simulink model "PFC_V11"  (R2016b)
settings: Solver=FixedStepDiscrete  StartTime=0.0  StopTime=0.1  FixedStep=.1e-6  RelTol=1e-3
libraries: powerlib x29, simulink x5
settings Model: Creator=a037702  LastModifiedBy=a037702

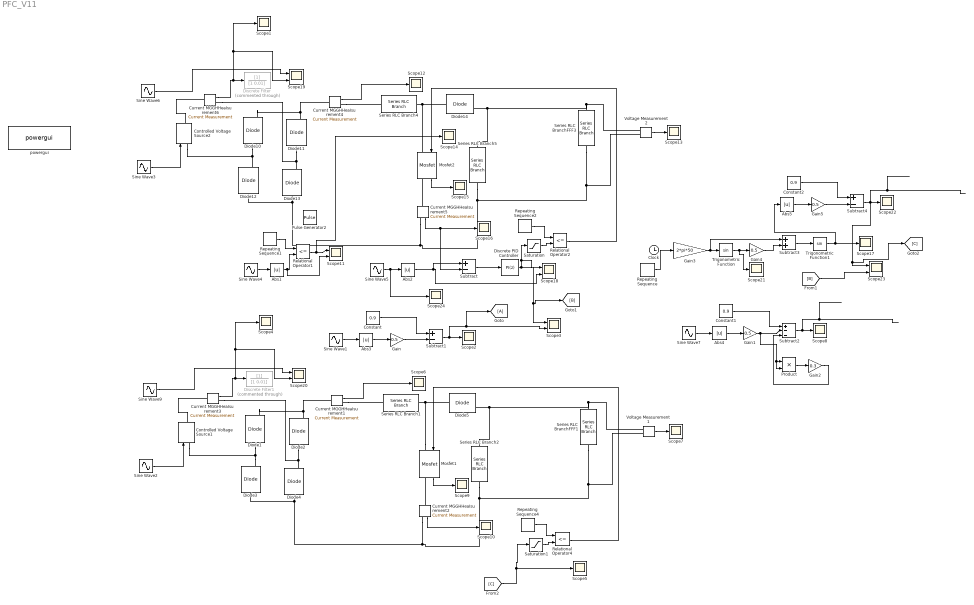
== system PFC_V11 ==
  Abs{1..5} (5 alike) : Abs
  Clock : Clock
  Constant : Constant  Value=0.9
  Constant1 : Constant  Value=0.9
  Constant2 : Constant  Value=0.9
  Controlled Voltage Source1 : powerlib/Electrical Sources/Controlled Voltage Source  Initialize=on  Source_Type=AC  Amplitude=0  Phase=0  Frequency=0  Measurements=None
  Controlled Voltage Source2 : powerlib/Electrical Sources/Controlled Voltage Source  Initialize=on  Source_Type=AC  Amplitude=0  Phase=0  Frequency=0  Measurements=None
  Current MGGHHeaIsurement{1..6} (6 alike) : powerlib/Measurements/Current Measurement  PhasorSimulation=off  OutputType=Complex  PSBequivalent=0
  Diode{1..5,10..14} (10 alike) : powerlib/Power Electronics/Diode  Ron=0.001  Lon=0  Vf=0.8  IC=0  UseSnubber=off  Rs=500  Cs=250e-9  Measurements=on
  Discrete Filter : DiscreteFilter  Commented=through  Denominator=[1 0.01]
  Discrete Filter1 : DiscreteFilter  Commented=through  Denominator=[1 0.01]
  Discrete PID Controller : simulink/Continuous/PID Controller  Controller=PI  TimeDomain=Discrete-time  SampleTime=-1  IntegratorMethod=Forward Euler  FilterMethod=Forward Euler  Form=Parallel  UseFilter=on  ControllerParametersSource=internal  P=0.001  I=100  D=0  N=100  InitialConditionSource=internal  InitialConditionForIntegrator=0  InitialConditionForFilter=0  ExternalReset=none  LimitOutput=off  UpperSaturationLimit=inf  LowerSaturationLimit=-inf  LinearizeAsGain=off  AntiWindupMode=none  Kb=1  TrackingMode=off  Kt=1  PParamMin=[]  PParamMax=[]  IParamMin=[]  IParamMax=[]  DParamMin=[]  DParamMax=[]  NParamMin=[]  NParamMax=[]  KbParamMin=[]  KbParamMax=[]  KtParamMin=[]  KtParamMax=[]  POutMin=[]  POutMax=[]  IOutMin=[]  IOutMax=[]  DOutMin=[]  DOutMax=[]  NOutMin=[]  NOutMax=[]  KbOutMin=[]  KbOutMax=[]  KtOutMin=[]  KtOutMax=[]  IntegratorOutMin=[]  IntegratorOutMax=[]  FilterOutMin=[]  FilterOutMax=[]  SumOutMin=[]  SumOutMax=[]  SumI1OutMin=[]  SumI1OutMax=[]  SumI2OutMin=[]  SumI2OutMax=[]  SumI3OutMin=[]  SumI3OutMax=[]  SumDOutMin=[]  SumDOutMax=[]  SaturationOutMin=[]  SaturationOutMax=[]  IntegratorContinuousStateAttributes=''  IntegratorStateMustResolveToSignalObject=off  IntegratorRTWStateStorageClass=Auto  FilterContinuousStateAttributes=''  FilterStateMustResolveToSignalObject=off  FilterRTWStateStorageClass=Auto  DifferentiatorICPrevScaledInput=0  DifferentiatorOutMin=[]  DifferentiatorOutMax=[]
  Gain{,1,4..5} (4 alike) : Gain  Gain=0.5
  Gain2 : Gain  Gain=0.3
  Gain3 : Gain  Gain=2*pi*50
  Mosfet1 : powerlib/Power Electronics/Mosfet  Ron=0.1  Lon=0  Rd=0.01  Vfd=0  IC=0  Rs=1e5  Cs=inf  Measurements=on
  Mosfet2 : powerlib/Power Electronics/Mosfet  Ron=0.1  Lon=0  Rd=0.01  Vfd=0  IC=0  Rs=1e5  Cs=inf  Measurements=on
  Product : Product
  Pulse Generator2 : DiscretePulseGenerator  PulseType=Time based  Amplitude=10  Period=10e-6  PulseWidth=50
  Relational Operator1 : RelationalOperator  Operator=<=  OutDataTypeStr=boolean  RndMeth=Simplest
  Relational Operator2 : RelationalOperator  Operator=<=  OutDataTypeStr=boolean  RndMeth=Simplest
  Relational Operator4 : RelationalOperator  Operator=<=  OutDataTypeStr=boolean  RndMeth=Simplest
  Repeating Sequence : simulink/Sources/Repeating Sequence  rep_seq_t=[0 0.01]  rep_seq_y=[0 0.01]
  Repeating Sequence1 : simulink/Sources/Repeating Sequence  rep_seq_t=[0 10e-6]  rep_seq_y=[0 1]
  Repeating Sequence2 : simulink/Sources/Repeating Sequence  rep_seq_t=[0 10e-6]  rep_seq_y=[0 1]
  Repeating Sequence4 : simulink/Sources/Repeating Sequence  rep_seq_t=[0 10e-6]  rep_seq_y=[0 1]
  Saturation : Saturate  UpperLimit=0.95  LowerLimit=0.05
  Saturation1 : Saturate  UpperLimit=0.95  LowerLimit=0.05
  Scope{1..2,4..10,12..17,21..22,24} (18 alike) : Scope
  Scope{3,11,18..20,23} (6 alike) : Scope  NumInputPorts=2
  Series RLC Branch1 : powerlib/Elements/Series RLC Branch  LConnTagsString=__new0  RConnTagsString=__new0  BranchType=L  Resistance=1  Inductance=500e-6  SetiL0=on  InitialCurrent=0  Capacitance=1e-6  Setx0=off  InitialVoltage=0  Measurements=Branch current
  Series RLC Branch2 : powerlib/Elements/Series RLC Branch  LConnTagsString=__new0  RConnTagsString=__new0  BranchType=R  Resistance=100  Inductance=500e-6  SetiL0=on  InitialCurrent=0  Capacitance=100e-6  Setx0=on  InitialVoltage=0  Measurements=Branch current
  Series RLC Branch4 : powerlib/Elements/Series RLC Branch  LConnTagsString=__new0  RConnTagsString=__new0  BranchType=L  Resistance=1  Inductance=500e-6  SetiL0=on  InitialCurrent=0  Capacitance=1e-6  Setx0=off  InitialVoltage=0  Measurements=Branch current
  Series RLC Branch5 : powerlib/Elements/Series RLC Branch  LConnTagsString=__new0  RConnTagsString=__new0  BranchType=R  Resistance=100  Inductance=500e-6  SetiL0=on  InitialCurrent=0  Capacitance=100e-6  Setx0=on  InitialVoltage=0  Measurements=Branch current
  Series RLC BranchFFF1 : powerlib/Elements/Series RLC Branch  LConnTagsString=__new0  RConnTagsString=__new0  BranchType=C  Resistance=1  Inductance=500e-6  SetiL0=on  InitialCurrent=0  Capacitance=100e-6  Setx0=on  InitialVoltage=0  Measurements=Branch current
  Series RLC BranchFFF3 : powerlib/Elements/Series RLC Branch  LConnTagsString=__new0  RConnTagsString=__new0  BranchType=C  Resistance=1  Inductance=500e-6  SetiL0=on  InitialCurrent=0  Capacitance=100e-6  Setx0=on  InitialVoltage=0  Measurements=Branch current
  Sine Wave1 : Sin  Frequency=2*pi*50  SampleTime=0
  Sine Wave2 : Sin  Amplitude=320  Frequency=2*pi*50  SampleTime=0
  Sine Wave3 : Sin  Amplitude=320  Frequency=2*pi*50  SampleTime=0
  Sine Wave4 : Sin  Amplitude=0.5  Frequency=2*pi*50  SampleTime=0
  Sine Wave5 : Sin  Amplitude=10  Frequency=2*pi*50  SampleTime=0
  Sine Wave6 : Sin  Amplitude=20  Frequency=2*pi*50  SampleTime=0
  Sine Wave7 : Sin  Frequency=2*pi*50  SampleTime=0
  Sine Wave9 : Sin  Amplitude=20  Frequency=2*pi*50  SampleTime=0
  Subtract : Sum  Inputs=+-
  Subtract1 : Sum  Inputs=+-
  Subtract2 : Sum  Inputs=+--
  Subtract3 : Sum
  Subtract4 : Sum  Inputs=+-
  Trigonometric Function : Trigonometry
  Trigonometric Function1 : Trigonometry
  Voltage Measurement1 : powerlib/Measurements/Voltage Measurement  PhasorSimulation=off  OutputType=Complex  PSBequivalent=0
  Voltage Measurement2 : powerlib/Measurements/Voltage Measurement  PhasorSimulation=off  OutputType=Complex  PSBequivalent=0
  powergui : powerlib/powergui  Priority=1  SimulationMode=Discrete  SolverType=Tustin/Backward Euler (TBE)  SampleTime=.1e-6  frequency=60  SPID=off  DisableSnubberDevices=off  DisableRonSwitches=off  DisableVfSwitches=off  SwTol=0  DisplayEquations=off  Interpol=off  ExternalGateDelay=off  methode=off  Ts=10  FunctionMessages=off  echomessages=off  HookPort=off  EnableUseOfTLC=off  x0status=blocks  frequencyindice=0  Pbase=100e6  ErrMax=1e-4  Iterations=50  UnitsV=kV  UnitsW=MW  buscounter=0  RestoreLinks=warning  ResistiveCurrentMeasurement=off  Frange=[0:2:500]  Ylog=off  Xlog=on  ShowGrid=off  save=off  variable=ZData  structure=0  ZoomFFT=off  StartTime=0.0  cycles=1  DisplayStyle=1  fundamental=60  FreqAxis=off  MaxFrequency=1000  frequencyindicesteady=1  RmsSteady=1  display=off
  wires:
  Sine Wave3/1 -> Controlled Voltage Source2/1
  Current MGGHHeaIsurement4/1 -> Scope12/1
  Voltage Measurement2/1 -> Scope13/1
  Relational Operator1/1 -> Scope14/1, Scope11/1
  Mosfet2/1 -> Scope15/1
  Current MGGHHeaIsurement5/1 -> Subtract/2, Scope16/1
  Sine Wave4/1 -> Abs1/1
  Repeating Sequence1/1 -> Relational Operator1/1
  Abs1/1 -> Scope11/2, Relational Operator1/2
  Sine Wave5/1 -> Scope24/1, Abs2/1
  Subtract/1 -> Discrete PID Controller/1
  Discrete PID Controller/1 -> [B], Scope3/1, Scope18/1, Saturation/1
  Saturation/1 -> Relational Operator2/2
  Repeating Sequence2/1 -> Relational Operator2/1
  Relational Operator2/1 -> Mosfet2/1
  Abs2/1 -> Scope18/2, Subtract/1
  Current MGGHHeaIsurement6/1 -> Scope19/2, Scope1/1, Discrete Filter/1
  Sine Wave6/1 -> Scope19/1
  Sine Wave1/1 -> Abs3/1
  Abs3/1 -> Gain/1
  Gain/1 -> Subtract1/2
  Constant/1 -> Subtract1/1
  Subtract1/1 -> [A], Scope3/2, Scope2/1
  Sine Wave2/1 -> Controlled Voltage Source1/1
  Current MGGHHeaIsurement1/1 -> Scope6/1
  Voltage Measurement1/1 -> Scope7/1
  Mosfet1/1 -> Scope9/1
  Current MGGHHeaIsurement2/1 -> Scope10/1
  Saturation1/1 -> Relational Operator4/2
  Repeating Sequence4/1 -> Relational Operator4/1
  Relational Operator4/1 -> Mosfet1/1
  Current MGGHHeaIsurement3/1 -> Scope20/2, Scope4/1, Discrete Filter1/1
  Sine Wave9/1 -> Scope20/1
  [C] -> Saturation1/1, Scope5/1
  Sine Wave7/1 -> Abs4/1
  Abs4/1 -> Gain1/1
  Gain1/1 -> Product/1, Product/2, Subtract2/2
  Constant1/1 -> Subtract2/1
  Subtract2/1 -> Scope8/1
  Product/1 -> Gain2/1
  Gain2/1 -> Subtract2/3
  Gain3/1 -> Subtract3/1, Trigonometric Function/1
  Repeating Sequence/1 -> Gain3/1
  Trigonometric Function/1 -> Scope21/1, Gain4/1
  Gain4/1 -> Subtract3/2
  Subtract3/1 -> Trigonometric Function1/1
  Trigonometric Function1/1 -> Abs5/1, Scope17/1
  Abs5/1 -> Gain5/1
  Gain5/1 -> Subtract4/2
  Constant2/1 -> Subtract4/1
  Subtract4/1 -> [C], Scope23/1, Scope22/1
  [B] -> Scope23/2
  connections:
  Diode11/RConn1 -- Diode10/RConn1 -- Current MGGHHeaIsurement4/LConn1
  Diode11/LConn1 -- Current MGGHHeaIsurement6/RConn1 -- Diode13/RConn1
  Diode10/LConn1 -- Controlled Voltage Source2/LConn1 -- Diode12/RConn1
  Diode13/LConn1 -- Current MGGHHeaIsurement5/RConn1 -- Series RLC Branch5/RConn1 -- Voltage Measurement2/LConn2 -- Series RLC BranchFFF3/RConn1 -- Diode12/LConn1
  Series RLC Branch4/RConn1 -- Diode14/LConn1 -- Mosfet2/LConn1
  Series RLC BranchFFF3/LConn1 -- Voltage Measurement2/LConn1 -- Series RLC Branch5/LConn1 -- Diode14/RConn1
  Current MGGHHeaIsurement4/RConn1 -- Series RLC Branch4/LConn1
  Current MGGHHeaIsurement5/LConn1 -- Mosfet2/RConn1
  Current MGGHHeaIsurement6/LConn1 -- Controlled Voltage Source2/RConn1
  Current MGGHHeaIsurement1/LConn1 -- Diode2/RConn1 -- Diode1/RConn1
  Diode4/RConn1 -- Diode2/LConn1 -- Current MGGHHeaIsurement3/RConn1
  Diode3/RConn1 -- Diode1/LConn1 -- Controlled Voltage Source1/LConn1
  Diode3/LConn1 -- Diode4/LConn1 -- Current MGGHHeaIsurement2/RConn1 -- Series RLC Branch2/RConn1 -- Voltage Measurement1/LConn2 -- Series RLC BranchFFF1/RConn1
  Mosfet1/LConn1 -- Series RLC Branch1/RConn1 -- Diode5/LConn1
  Diode5/RConn1 -- Series RLC Branch2/LConn1 -- Series RLC BranchFFF1/LConn1 -- Voltage Measurement1/LConn1
  Current MGGHHeaIsurement1/RConn1 -- Series RLC Branch1/LConn1
  Current MGGHHeaIsurement3/LConn1 -- Controlled Voltage Source1/RConn1
  Current MGGHHeaIsurement2/LConn1 -- Mosfet1/RConn1
